simulink model "PneumaticsSystem"  (R2019b)
settings: configuration reference "ConfigSet_PneumaticsSystem_Reference" (kept outside this file)
PostLoadFcn:
  | set_up_test_model()
model workspace (MAT data in the model file):
  PAtm = 101300
  Prm_PneumaticsSystem : Simulink.Parameter (value not decoded)
  SampleTime = 0.01
symbols that are objects in the model workspace (value not decoded): Prm_PneumaticsSystem
undefined symbols (not defined in the file): AirSuspensionBogie1Deflated, AirSuspensionPressure, AirSuspensionPressureSwitch, AirSuspPressureDiff, AuxiliaryReservoirPressure, AuxiliaryReservoirPressureSwitch, BECU1BrakeNotApplied, BECU1BrakeNotReleased, BECU1CarLoadPressureLow, BECU1EmergencyBrakeFailure, BECU1LoadPressureLow, BECU1ServiceBrakeFailure, BECU2CarLoadPressureLow, BECU2EmergencyBrakeFailure, BECULowRPressure, Bogie, BrakeCylinderControlPressure, BrakeCylinderPressure, BrakeCylinderPressureGauge, BrakeCylinderPressureSwitch, BrakeReservoirPressure, BrakeReservoirPressureSwitch, HornHighPressureSwitch, HornLowPressureSwitch, MainReservoirPipePressure, MainReservoirPipePressureSwitch, MainReservoirPressure, MainReservoirPressureGauge, MainReservoirPressureSwitch, MaxAxles, MRPS_TractionCutout, ORDPressureSwitch, PantographCylinderPressure, ParkBrakePressure, ParkBrakePressureGauge, ParkBrakePressureSwitch, PS2, PS3, SandingSystemPressure, SandingSystemPressureSwitch, SRPressureGauge, VCBCylinderPressure, VCBPressureSwitch
libraries: PneumaticLib x56, simulink x50, LatchesLib x7, FiltersLib x4, TimersLib x3, MathOperationsLib x3, VectorOperationsLib x1, simulink_extras x1
(part 2 of 3)

== system PneumaticsSystem/PneumaticsPerVehicle/PneumaticsSystem/AuxiliarySystems/Horn ==
  ControlStates : Inport
  HornSupplyPressure : Inport  Port=2
  ElectricalSignals : Inport  Port=3
  Enable : EnablePort
  Bias : Bias  Bias=-PAtm
  Bus Creator : BusCreator  Inputs=2
  Bus Creator1 : BusCreator  Inputs=2
  Bus Selector : BusSelector  OutputSignals=HornLowIsolationCock,HornHighIsolationCock
  Bus Selector1 : BusSelector  OutputSignals=HornLowControl,HornHighControl,RemoteHornIsolate
  Data Type Conversion : DataTypeConversion
  Data Type Conversion1 : DataTypeConversion
  Enough Air : simulink/Logic and Bit Operations/Compare To Constant  relop=>  const=PressureSwitchON  OutDataTypeStr=boolean
  Enough Air1 : simulink/Logic and Bit Operations/Compare To Constant  relop=>  const=PressureSwitchON  OutDataTypeStr=boolean
  Gain : Gain
  Gain1 : Gain
  High Horn : simulink/Logic and Bit Operations/Compare To Constant  relop===  const=1  OutDataTypeStr=boolean
  Logical Operator : Logic  Inputs=3  AllPortsSameDT=off  OutDataTypeStr=boolean
  Logical Operator1 : Logic  Inputs=3  AllPortsSameDT=off  OutDataTypeStr=boolean
  Low Horn : simulink/Logic and Bit Operations/Compare To Constant  relop===  const=1  OutDataTypeStr=boolean
  NOT : Logic  Operator=NOT  AllPortsSameDT=off  OutDataTypeStr=boolean
  Product : Product
  Product1 : Product
  PressureSwitches : Outport
  AudioOut : Outport  Port=2
  wires:
  ControlStates/1 -> Bus Selector/1
  Bus Selector1/1 -> High Horn/1  "<HornLowControl>"
  Bias/1 -> Product1/2, Product/2
  Product/1 -> Enough Air/1
  High Horn/1 -> Logical Operator/1
  Low Horn/1 -> Logical Operator1/1
  Logical Operator/1 -> Data Type Conversion/1  "HornLowPressureSwitch"
  Logical Operator1/1 -> Data Type Conversion1/1  "HornHighPressureSwitch"
  Gain/1 -> Bus Creator/1  "HornLow"
  Gain1/1 -> Bus Creator/2  "HornHigh"
  Bus Creator/1 -> AudioOut/1
  Bus Creator1/1 -> PressureSwitches/1  "HornPressureSwitches"
  Data Type Conversion/1 -> Gain/1, Bus Creator1/1  "HornLowPressureSwitch"
  Data Type Conversion1/1 -> Gain1/1, Bus Creator1/2  "HornHighPressureSwitch"
  HornSupplyPressure/1 -> Bias/1
  ElectricalSignals/1 -> Bus Selector1/1
  Bus Selector/1 -> Product1/1  "<HornLowIsolationCock>"
  Bus Selector1/3 -> NOT/1  "<RemoteHornIsolate>"
  NOT/1 -> Logical Operator1/3, Logical Operator/3
  Bus Selector1/2 -> Low Horn/1  "<HornHighControl>"
  Product1/1 -> Enough Air1/1
  Enough Air1/1 -> Logical Operator/2
  Bus Selector/2 -> Product/1  "<HornHighIsolationCock>"
  Enough Air/1 -> Logical Operator1/2

== system PneumaticsSystem/PneumaticsPerVehicle/PneumaticsSystem/BogiePneumaticSystems/AirSuspensionSystem ==
  Faults : Inport
  ControlStates : Inport  Port=2
  PhysicalSignals : Inport  Port=3
  AirSuspensionSupplyPressure : Inport  Port=4
  Reset : Inport  Port=5
  Enable : EnablePort
  AirSuspensionPerBogie : Subsystem
  Bus Selector1 : BusSelector  OutputSignals=BogieSupportedMasses
  Bus Selector3 : BusSelector  OutputSignals=AirSuspensionSystemIsolationCockBogie1,AirSuspensionSystemIsolationCockBogie2,AirSuspensionSystemDrainCockBogie1,AirSuspensionSystemDrainCockBogie2
  Sum : Sum  Inputs=1
  Terminator : Terminator
  Vector Concatenate1 : Concatenate
  Vector Concatenate2 : Concatenate
  AirSuspensionPressure : Outport
  ASPressureSwitches : Outport  Port=2
  AirSuspPressure%Variation : Outport  Port=3
  ASRToAS : Outport  Port=4
  wires:
  ControlStates/1 -> Bus Selector3/1
  AirSuspensionPerBogie/1(AirSuspensionPressure) -> AirSuspensionPressure/1
  Bus Selector3/1 -> Vector Concatenate2/1  "<AirSuspensionSystemIsolationCockBogie1>"
  Reset/1 -> AirSuspensionPerBogie/5(Reset)
  Vector Concatenate1/1 -> AirSuspensionPerBogie/3(AirSuspensionDrainCock)
  PhysicalSignals/1 -> Bus Selector1/1
  Bus Selector3/2 -> Vector Concatenate2/2  "<AirSuspensionSystemIsolationCockBogie2>"
  Vector Concatenate2/1 -> AirSuspensionPerBogie/2(AirSuspensionIsolCock)
  AirSuspensionSupplyPressure/1 -> AirSuspensionPerBogie/1(AirSuspensionSupplyPressure)
  AirSuspensionPerBogie/3(AirSuspensionPressureSwitch) -> ASPressureSwitches/1
  Bus Selector1/1 -> AirSuspensionPerBogie/4(BogieSupportedMass)  "<BogieSupportedMasses>"
  Bus Selector3/3 -> Vector Concatenate1/1  "<AirSuspensionSystemDrainCockBogie1>"
  Bus Selector3/4 -> Vector Concatenate1/2  "<AirSuspensionSystemDrainCockBogie2>"
  AirSuspensionPerBogie/2(AirSuspensionValve) -> Terminator/1
  Faults/1 -> AirSuspensionPerBogie/6(Faults)
  AirSuspensionPerBogie/4(AirSuspPressure%Variation) -> AirSuspPressure%Variation/1
  AirSuspensionPerBogie/5(ASRToAS) -> Sum/1
  Sum/1 -> ASRToAS/1

== system PneumaticsSystem/PneumaticsPerVehicle/PneumaticsSystem/BogiePneumaticSystems/BogiePressureMapping ==
  BrakeControlPressures : Inport  Partition=on  PartitionDimension=1  PartitionWidth=1  PartitionOffset=0
  BrakeCylinderPressures : Inport  Port=2  Partition=on  PartitionDimension=1  PartitionWidth=2  PartitionOffset=0
  ParkBrakePressures : Inport  Port=3  Partition=on  PartitionDimension=1  PartitionWidth=1  PartitionOffset=0
  AirSuspensionPressures : Inport  Port=4  Partition=on  PartitionDimension=1  PartitionWidth=1  PartitionOffset=0
  SandingPressures : Inport  Port=5  Partition=on  PartitionDimension=1  PartitionWidth=1  PartitionOffset=0
  AirSuspPressure%Variation : Inport  Port=6  Partition=on  PartitionDimension=1  PartitionWidth=1  PartitionOffset=0
  Bus Assignment : BusAssignment  AssignedSignals=BrakeCylinderControlPressure,BrakeCylinderPressure,ParkBrakePressure,SandingSystemPressure,AirSuspensionPressure,AirSuspPressureDiff
  Constant : Constant  Value=0  OutDataTypeStr=Bus: BD_PneumaticsSystem_Out_Vehicle_Debug_Bogie
  For Each : ForEach  DisableCoverage=on
  BogiePressures : Outport  ConcatenationDimension=1
  wires:
  BrakeCylinderPressures/1 -> Bus Assignment/3
  Constant/1 -> Bus Assignment/1
  Bus Assignment/1 -> BogiePressures/1  "Debug"
  ParkBrakePressures/1 -> Bus Assignment/4
  AirSuspensionPressures/1 -> Bus Assignment/6
  SandingPressures/1 -> Bus Assignment/5
  BrakeControlPressures/1 -> Bus Assignment/2
  AirSuspPressure%Variation/1 -> Bus Assignment/7

== system PneumaticsSystem/PneumaticsPerVehicle/PneumaticsSystem/BogiePneumaticSystems/BogiePressureSwitchesMapping ==
  BrakeCylinderPressureSwitches : Inport  Partition=on  PartitionDimension=1  PartitionWidth=1  PartitionOffset=0
  ParkBrakePressureSwitches : Inport  Port=2  Partition=on  PartitionDimension=1  PartitionWidth=1  PartitionOffset=0
  AirSuspensionPressureSwitches : Inport  Port=3  Partition=on  PartitionDimension=1  PartitionWidth=1  PartitionOffset=0
  SandingPressureSwitches : Inport  Port=4  Partition=on  PartitionDimension=1  PartitionWidth=1  PartitionOffset=0
  Bus Assignment : BusAssignment  AssignedSignals=BrakeCylinderPressureSwitch,ParkBrakePressureSwitch,AirSuspensionPressureSwitch,SandingSystemPressureSwitch
  Constant : Constant  Value=0  OutDataTypeStr=Bus: BD_PneumaticsSystem_Out_Vehicle_Switches_Bogie
  For Each : ForEach  DisableCoverage=on
  BogiePressureSwitches : Outport  ConcatenationDimension=1
  wires:
  SandingPressureSwitches/1 -> Bus Assignment/5
  AirSuspensionPressureSwitches/1 -> Bus Assignment/4
  Bus Assignment/1 -> BogiePressureSwitches/1
  Constant/1 -> Bus Assignment/1
  ParkBrakePressureSwitches/1 -> Bus Assignment/3
  BrakeCylinderPressureSwitches/1 -> Bus Assignment/2

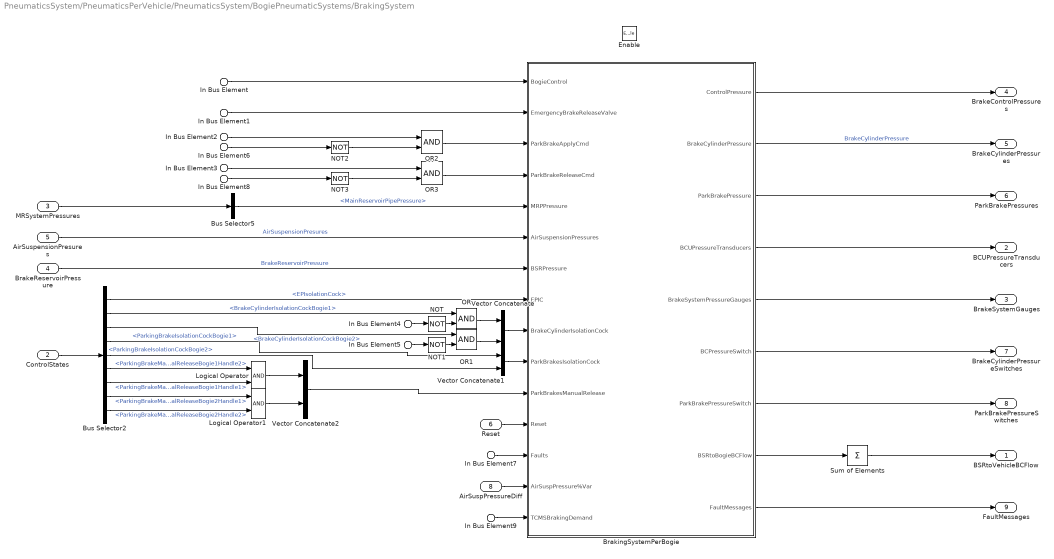
== system PneumaticsSystem/PneumaticsPerVehicle/PneumaticsSystem/BogiePneumaticSystems/BrakingSystem ==
  In Bus Element : Inport  PortName=ElectricalSignals  Element=BogieControl
  In Bus Element1 : Inport  PortName=ElectricalSignals  Element=NoEmergencyBrakeValve
  In Bus Element2 : Inport  PortName=ElectricalSignals  Element=ParkingBrakeApplyCmd
  In Bus Element3 : Inport  PortName=ElectricalSignals  Element=ParkingBrakeReleaseCmd
  In Bus Element9 : Inport  PortName=ElectricalSignals  Element=TCMSBrakingDemand
  In Bus Element4 : Inport  PortName=ElectricalSignals  Element=RemoteMagnetValve1
  In Bus Element5 : Inport  PortName=ElectricalSignals  Element=RemoteMagnetValve2
  ControlStates : Inport  Port=2
  MRSystemPressures : Inport  Port=3
  BrakeReservoirPressure : Inport  Port=4
  AirSuspensionPresures : Inport  Port=5
  Reset : Inport  Port=6
  In Bus Element7 : Inport  Port=7  PortName=PneumaticsFaults
  In Bus Element6 : Inport  Port=7  PortName=PneumaticsFaults  Element=ParkingBrakeApplicationFailure
  In Bus Element8 : Inport  Port=7  PortName=PneumaticsFaults  Element=ParkingBrakeReleaseFailure
  AirSuspPressureDiff : Inport  Port=8
  Enable : EnablePort
  BrakingSystemPerBogie : Subsystem
  Bus Selector2 : BusSelector  OutputSignals=EPIsolationCock,BrakeCylinderIsolationCockBogie1,BrakeCylinderIsolationCockBogie2,ParkingBrakeIsolationCockBogie1,ParkingBrakeIsolationCockBogie2,ParkingBrakeManualReleaseBogie1Handle2,ParkingBrakeManualReleaseBogie1Handle1,ParkingBrakeManualReleaseBogie2Handle1,ParkingBrakeManualReleaseBogie2Handle2
  Bus Selector5 : BusSelector  OutputSignals=MainReservoirPipePressure
  Logical Operator : Logic  AllPortsSameDT=off  OutDataTypeStr=boolean
  Logical Operator1 : Logic  AllPortsSameDT=off  OutDataTypeStr=boolean
  NOT{,1..3} (4 alike) : Logic  Operator=NOT  AllPortsSameDT=off  OutDataTypeStr=boolean
  OR{,1..3} (4 alike) : Logic  AllPortsSameDT=off  OutDataTypeStr=boolean
  Sum of Elements : Sum  Inputs=+
  Vector Concatenate : Concatenate
  Vector Concatenate1 : Concatenate
  Vector Concatenate2 : Concatenate
  BSRtoVehicleBCFlow : Outport
  BCUPressureTransducers : Outport  Port=2
  BrakeSystemGauges : Outport  Port=3
  BrakeControlPressures : Outport  Port=4
  BrakeCylinderPressures : Outport  Port=5
  ParkBrakePressures : Outport  Port=6
  BrakeCylinderPressureSwitches : Outport  Port=7
  ParkBrakePressureSwitches : Outport  Port=8
  FaultMessages : Outport  Port=9
  wires:
  BrakingSystemPerBogie/1(ControlPressure) -> BrakeControlPressures/1
  In Bus Element/1 -> BrakingSystemPerBogie/1(BogieControl)
  In Bus Element1/1 -> BrakingSystemPerBogie/2(EmergencyBrakeReleaseValve)
  BrakeReservoirPressure/1 -> BrakingSystemPerBogie/7(BSRPressure)  "BrakeReservoirPressure"
  ControlStates/1 -> Bus Selector2/1
  AirSuspensionPresures/1 -> BrakingSystemPerBogie/6("AirSuspensionPressures ")  "AirSuspensionPresures"
  BrakingSystemPerBogie/2(BrakeCylinderPressure) -> BrakeCylinderPressures/1  "BrakeCylinderPressure"
  BrakingSystemPerBogie/8(BSRtoBogieBCFlow) -> Sum of Elements/1
  Bus Selector5/1 -> BrakingSystemPerBogie/5(MRPPressure)  "<MainReservoirPipePressure>"
  BrakingSystemPerBogie/5(BrakeSystemPressureGauges) -> BrakeSystemGauges/1
  BrakingSystemPerBogie/7(ParkBrakePressureSwitch) -> ParkBrakePressureSwitches/1
  BrakingSystemPerBogie/3(ParkBrakePressure) -> ParkBrakePressures/1
  BrakingSystemPerBogie/4(BCUPressureTransducers) -> BCUPressureTransducers/1
  MRSystemPressures/1 -> Bus Selector5/1
  BrakingSystemPerBogie/6(BCPressureSwitch) -> BrakeCylinderPressureSwitches/1
  Reset/1 -> BrakingSystemPerBogie/12(Reset)
  Sum of Elements/1 -> BSRtoVehicleBCFlow/1
  Bus Selector2/6 -> Logical Operator/1  "<ParkingBrakeManualReleaseBogie1Handle2>"
  Bus Selector2/7 -> Logical Operator/2  "<ParkingBrakeManualReleaseBogie1Handle1>"
  Vector Concatenate2/1 -> BrakingSystemPerBogie/11(ParkBrakesManualRelease)
  In Bus Element2/1 -> OR2/1
  In Bus Element3/1 -> OR3/1
  Bus Selector2/8 -> Logical Operator1/1  "<ParkingBrakeManualReleaseBogie2Handle1>"
  Bus Selector2/9 -> Logical Operator1/2  "<ParkingBrakeManualReleaseBogie2Handle2>"
  Logical Operator/1 -> Vector Concatenate2/1
  Logical Operator1/1 -> Vector Concatenate2/2
  In Bus Element7/1 -> BrakingSystemPerBogie/13(Faults)
  OR2/1 -> BrakingSystemPerBogie/3(ParkBrakeApplyCmd)
  OR3/1 -> BrakingSystemPerBogie/4(ParkBrakeReleaseCmd)
  NOT2/1 -> OR2/2
  In Bus Element6/1 -> NOT2/1
  NOT3/1 -> OR3/2
  In Bus Element8/1 -> NOT3/1
  BrakingSystemPerBogie/9(FaultMessages) -> FaultMessages/1
  AirSuspPressureDiff/1 -> BrakingSystemPerBogie/14(AirSuspPressure%Var)
  Bus Selector2/1 -> BrakingSystemPerBogie/8(EPIC)  "<EPIsolationCock>"
  In Bus Element9/1 -> BrakingSystemPerBogie/15(TCMSBrakingDemand)
  Vector Concatenate/1 -> BrakingSystemPerBogie/9(BrakeCylinderIsolationCock)
  Bus Selector2/4 -> Vector Concatenate1/1  "<ParkingBrakeIsolationCockBogie1>"
  OR/1 -> Vector Concatenate/1
  NOT1/1 -> OR1/2
  In Bus Element5/1 -> NOT1/1
  Bus Selector2/3 -> OR1/1  "<BrakeCylinderIsolationCockBogie2>"
  Bus Selector2/5 -> Vector Concatenate1/2  "<ParkingBrakeIsolationCockBogie2>"
  In Bus Element4/1 -> NOT/1
  NOT/1 -> OR/2
  OR1/1 -> Vector Concatenate/2
  Bus Selector2/2 -> OR/1  "<BrakeCylinderIsolationCockBogie1>"
  Vector Concatenate1/1 -> BrakingSystemPerBogie/10(ParkBrakesIsolationCock)

== system PneumaticsSystem/PneumaticsPerVehicle/PneumaticsSystem/BogiePneumaticSystems/SandingSystem ==
  ElectricalSignals : Inport
  ControlStates : Inport  Port=2
  SandingSystemSupplyPressure : Inport  Port=3
  Enable : EnablePort
  Bus Selector1 : BusSelector  OutputSignals=SandingSystemIsolationCockBogie1,SandingSystemIsolationCockBogie2
  Bus Selector2 : BusSelector  OutputSignals=SandingValve
  SandingSystemPerBogie : Subsystem
  Vector Concatenate : Concatenate
  SandingPressures : Outport
  SandingPressureSwitches : Outport  Port=2
  wires:
  ElectricalSignals/1 -> Bus Selector2/1
  ControlStates/1 -> Bus Selector1/1
  Bus Selector1/1 -> Vector Concatenate/1  "<SandingSystemIsolationCockBogie1>"
  Bus Selector1/2 -> Vector Concatenate/2  "<SandingSystemIsolationCockBogie2>"
  Vector Concatenate/1 -> SandingSystemPerBogie/1(SandingSystemIsolationCock)  "SandingSystemIsolationCock"
  SandingSystemSupplyPressure/1 -> SandingSystemPerBogie/2(SandingSystemSupplyPressure)
  Bus Selector2/1 -> SandingSystemPerBogie/3(SandingValve)  "<SandingValve>"
  SandingSystemPerBogie/1(SandingPressure) -> SandingPressures/1
  SandingSystemPerBogie/2(SandingPressureSwitch) -> SandingPressureSwitches/1

== system PneumaticsSystem/PneumaticsPerVehicle/PneumaticsSystem/BrakeReservoirSystem/BrakeSupplyReservoir ==
  MRPPressure : Inport
  BSRIsolCock : Inport  Port=2
  BSRDrainCock : Inport  Port=3
  BSRtoBCFlow : Inport  Port=4
  LowRPress : Inport  Port=5
  Reset : Inport  Port=6
  Preset : Inport  Port=7
  PresetVal : Inport  Port=8
  Enable : EnablePort
  BSRPressureSwitch.05 : PneumaticLib/Pressure Switch  OnSwitchValue=PressureSwitchON  OffSwitchValue=PressureSwitchOFF  OnOutputValue=1  OffOutputValue=0  InitOn=on
      settings: SourceProductName=Train Library
  Bias : Bias  Bias=-PAtm
  BrakeSupplyReservoir : PneumaticLib/Limited Air Pressure Vessel  resetPrs=ResetPressure + PAtm
      settings: SourceProductName=Pneumatic
  Constant : Constant  Value=PAtm + MaxPressure
  Display : Display
  FlowCalc : Subsystem
  Terminator : Terminator
  Unit Delay : UnitDelay  SampleTime=-1  HasFrameUpgradeWarning=on
  pAtm : Constant  Value=PAtm
  pAtm2 : Constant  Value=Volume
  BSRPressure : Outport
  BSRPressureSwitch : Outport  Port=2
  MRPToBSR : Outport  Port=3
  BSRPressureGauge : Outport  Port=4
  wires:
  pAtm2/1 -> BrakeSupplyReservoir/2
  pAtm/1 -> BrakeSupplyReservoir/4
  Reset/1 -> BrakeSupplyReservoir/5
  Unit Delay/1 -> FlowCalc/2(BSRPressure)
  MRPPressure/1 -> FlowCalc/1(MRPressure)
  Constant/1 -> BrakeSupplyReservoir/3
  FlowCalc/2(Flow) -> BrakeSupplyReservoir/1
  BrakeSupplyReservoir/1 -> BSRPressure/1, Bias/1, Unit Delay/1
  BrakeSupplyReservoir/2 -> Terminator/1
  BSRIsolCock/1 -> FlowCalc/3(BSRIsolCock)
  BSRtoBCFlow/1 -> FlowCalc/5(BSRtoBCFlow)
  BSRDrainCock/1 -> FlowCalc/4(BSRDrainCock)
  BSRPressureSwitch.05/1 -> BSRPressureSwitch/1  "BrakeReservoirPressureSwitch"
  Bias/1 -> BSRPressureGauge/1, Display/1, BSRPressureSwitch.05/1
  PresetVal/1 -> BrakeSupplyReservoir/7
  Preset/1 -> BrakeSupplyReservoir/6
  LowRPress/1 -> FlowCalc/6(Fault)
  FlowCalc/1(MRPToBSR) -> MRPToBSR/1

== system PneumaticsSystem/PneumaticsPerVehicle/PneumaticsSystem/GaugesMapping/Subsystem ==
  BCPressure : Inport  Partition=on  PartitionDimension=1  PartitionWidth=1  PartitionOffset=0
  Bus Assignment1 : BusAssignment  AssignedSignals=BrakeCylinderPressureGauge,ParkBrakePressureGauge
  Bus Selector : BusSelector  OutputSignals=BrakeCylinderPressureGauge,ParkBrakePressureGauge
  Constant1 : Constant  Value=0  OutDataTypeStr=Bus: BD_PneumaticsSystem_Out_Vehicle_Gauges_Bogie
  For Each : ForEach  DisableCoverage=on
  Bogie : Outport  ConcatenationDimension=1
  wires:
  Constant1/1 -> Bus Assignment1/1
  Bus Assignment1/1 -> Bogie/1  "Bogie"
  Bus Selector/1 -> Bus Assignment1/2  "<BrakeCylinderPressureGauge>"
  BCPressure/1 -> Bus Selector/1
  Bus Selector/2 -> Bus Assignment1/3  "<ParkBrakePressureGauge>"

== system PneumaticsSystem/PneumaticsPerVehicle/PneumaticsSystem/MainReservoirSystem/MainReservoir ==
  note: This pressure switch is not a part of
      | schematics and not used anywhere.
  CompressorRunning : Inport
  AirSupplyIsolationCock : Inport  Port=2
  MainReservoirIsolationCock : Inport  Port=3
  MainReservoirDrainCock : Inport  Port=4
  MRPPressure : Inport  Port=5
  Coupled : Inport  Port=6
  Reset : Inport  Port=7
  Enable : EnablePort
  Bias : Bias  Bias=-PAtm
  Constant : Constant  Value=PAtm + MaxPressure
  Display : Display
  FlowCalc : Subsystem
  Ground2 : Ground
  MRPressureSwitch.06 : PneumaticLib/Pressure Switch  OnSwitchValue=PressureSwitchON  OffSwitchValue=PressureSwitchOFF  OnOutputValue=1  OffOutputValue=0  InitOn=on
      settings: SourceProductName=Train Library
  MainReservoir : PneumaticLib/Limited Air Pressure Vessel  resetPrs=ResetPressure + PAtm
      settings: SourceProductName=Pneumatic
  Terminator : Terminator
  Unit Delay : UnitDelay  SampleTime=-1  HasFrameUpgradeWarning=on
  Vol : Constant  Value=Volume
  pAtm : Constant  Value=PAtm
  MRPressure : Outport
  MRPressureSwitch : Outport  Port=2
  MRPToMRFlow : Outport  Port=3
  wires:
  MainReservoir/2 -> Terminator/1
  FlowCalc/2(Flow) -> MainReservoir/1
  MainReservoir/1 -> MRPressure/1, Bias/1, Unit Delay/1  "MainReservoirPressure"
  Constant/1 -> MainReservoir/3
  MRPPressure/1 -> FlowCalc/6(MRPPressure)
  Unit Delay/1 -> FlowCalc/7(MRPressure)
  Reset/1 -> MainReservoir/5
  pAtm/1 -> MainReservoir/4
  Ground2/1 -> MainReservoir/6, MainReservoir/7
  Vol/1 -> MainReservoir/2
  CompressorRunning/1 -> FlowCalc/1(CompressorRunning)
  AirSupplyIsolationCock/1 -> FlowCalc/2(AirSupplyIsolCock)
  MainReservoirIsolationCock/1 -> FlowCalc/3(MRIsolCock)
  MainReservoirDrainCock/1 -> FlowCalc/4(MRDrainCock)
  MRPressureSwitch.06/1 -> MRPressureSwitch/1  "MainReservoirPressureSwitch"
  Bias/1 -> MRPressureSwitch.06/1, Display/1
  FlowCalc/1(MRPToMRFlow) -> MRPToMRFlow/1
  Coupled/1 -> FlowCalc/5(Coupled)

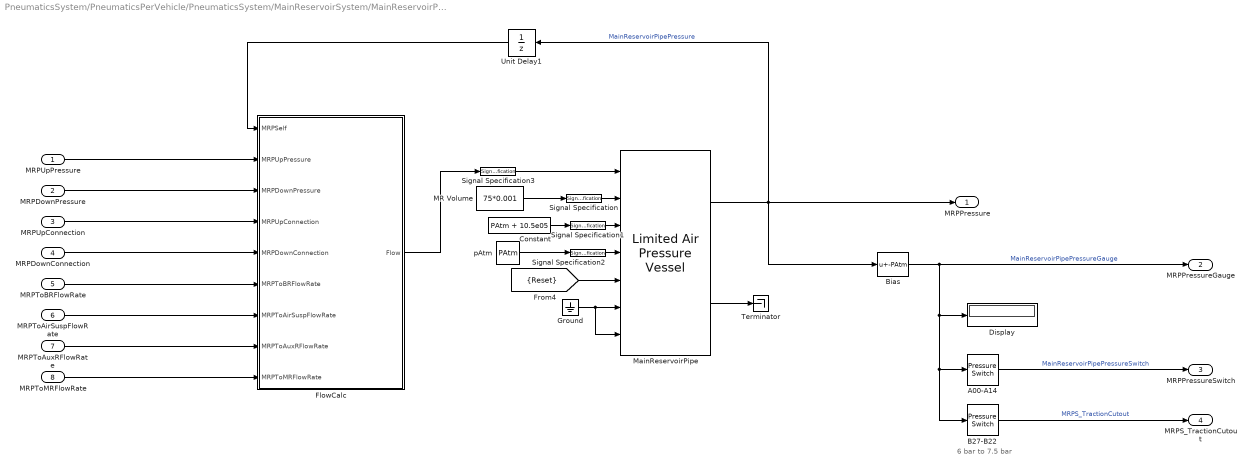
== system PneumaticsSystem/PneumaticsPerVehicle/PneumaticsSystem/MainReservoirSystem/MainReservoirPipe ==
  note: 6 bar to 7.5 bar
  MRPUpPressure : Inport
  MRPDownPressure : Inport  Port=2
  MRPUpConnection : Inport  Port=3
  MRPDownConnection : Inport  Port=4
  MRPToBRFlowRate : Inport  Port=5
  MRPToAirSuspFlowRate : Inport  Port=6
  MRPToAuxRFlowRate : Inport  Port=7
  MRPToMRFlowRate : Inport  Port=8
  A00-A14 : PneumaticLib/Pressure Switch  OnSwitchValue=PressureSwitchON  OffSwitchValue=PressureSwitchOFF  OnOutputValue=1  OffOutputValue=0  InitOn=on
      settings: SourceProductName=Train Library
  B27-B22 : PneumaticLib/Pressure Switch  OnSwitchValue=7e5  OffSwitchValue=6e5  OnOutputValue=1  OffOutputValue=0  InitOn=on
      settings: SourceProductName=Train Library
  Bias : Bias  Bias=-PAtm
  Constant : Constant  Value=PAtm + 10.5e05
  Display : Display
  FlowCalc : Subsystem
  Ground : Ground
  MR Volume : Constant  Value=75*0.001
  MainReservoirPipe : PneumaticLib/Limited Air Pressure Vessel  resetPrs=ResetPressure + PAtm
      settings: SourceProductName=Pneumatic
  Signal Specification : SignalSpecification  Unit=m^3
  Signal Specification1 : SignalSpecification  Unit=Pa
  Signal Specification2 : SignalSpecification  Unit=Pa
  Signal Specification3 : SignalSpecification  Unit=kg/s
  Terminator : Terminator
  Unit Delay1 : UnitDelay  SampleTime=-1  HasFrameUpgradeWarning=on
  pAtm : Constant  Value=PAtm
  MRPPressure : Outport  VectorParamsAs1DForOutWhenUnconnected=off
  MRPPressureGauge : Outport  Port=2
  MRPPressureSwitch : Outport  Port=3
  MRPS_TractionCutout : Outport  Port=4
  wires:
  MRPToBRFlowRate/1 -> FlowCalc/6(MRPToBRFlowRate)
  [Reset] -> MainReservoirPipe/5
  MRPToAirSuspFlowRate/1 -> FlowCalc/7(MRPToAirSuspFlowRate)
  Unit Delay1/1 -> FlowCalc/1(MRPSelf)
  Signal Specification2/1 -> MainReservoirPipe/4
  MRPToMRFlowRate/1 -> FlowCalc/9(MRPToMRFlowRate)
  Signal Specification/1 -> MainReservoirPipe/2
  MainReservoirPipe/2 -> Terminator/1
  Signal Specification3/1 -> MainReservoirPipe/1
  pAtm/1 -> Signal Specification2/1
  MR Volume/1 -> Signal Specification/1
  Constant/1 -> Signal Specification1/1
  FlowCalc/1(Flow) -> Signal Specification3/1
  MRPDownPressure/1 -> FlowCalc/3(MRPDownPressure)
  MRPUpPressure/1 -> FlowCalc/2(MRPUpPressure)
  MRPDownConnection/1 -> FlowCalc/5(MRPDownConnection)
  Signal Specification1/1 -> MainReservoirPipe/3
  MRPUpConnection/1 -> FlowCalc/4(MRPUpConnection)
  MainReservoirPipe/1 -> Bias/1, Unit Delay1/1, MRPPressure/1  "MainReservoirPipePressure"
  A00-A14/1 -> MRPPressureSwitch/1  "MainReservoirPipePressureSwitch"
  Bias/1 -> A00-A14/1, B27-B22/1, Display/1, MRPPressureGauge/1  "MainReservoirPipePressureGauge"
  B27-B22/1 -> MRPS_TractionCutout/1  "MRPS_TractionCutout"
  MRPToAuxRFlowRate/1 -> FlowCalc/8(MRPToAuxRFlowRate)
  Ground/1 -> MainReservoirPipe/7, MainReservoirPipe/6

== system PneumaticsSystem/PneumaticsPerVehicle/PneumaticsSystem/ASReservoir/Air SuspensionReservoir/FlowCalc ==
  MRPressure : Inport
  ASRPressure : Inport  Port=2
  ASRIsolCock : Inport  Port=3
  ASRDrainCock : Inport  Port=4
  ASFlow : Inport  Port=5
  Add : Sum  Inputs=+---
  BSR Charge : PneumaticLib/SS One Way Valve  d=0.015  p_deadband=1000
      settings: SourceProductName=Train Library
  BSR Vent Drain : PneumaticLib/SS One Way Valve  d=0.015  p_deadband=1000
      settings: SourceProductName=Train Library
  BSR Vent IC : PneumaticLib/SS One Way Valve  d=0.015  p_deadband=1000
      settings: SourceProductName=Train Library
  Compare To Constant : simulink/Logic and Bit Operations/Compare To Constant  relop=>=  const=780000  OutDataTypeStr=boolean
  Constant : Constant  Value=PAtm
  Logical Operator1 : Logic  Operator=NOT  AllPortsSameDT=off  OutDataTypeStr=boolean
  Logical Operator2 : Logic  Operator=NOT  AllPortsSameDT=off  OutDataTypeStr=boolean
  Logical Operator3 : Logic  Operator=OR  AllPortsSameDT=off  OutDataTypeStr=boolean
  Terminator : Terminator
  Terminator1 : Terminator
  Terminator4 : Terminator
  MRPToASR : Outport
  Flow : Outport  Port=2
  wires:
  Logical Operator2/1 -> BSR Vent Drain/3
  ASFlow/1 -> Add/4
  ASRDrainCock/1 -> Logical Operator2/1
  BSR Vent Drain/1 -> Add/3
  BSR Vent Drain/2 -> Terminator4/1
  ASRPressure/1 -> Compare To Constant/1, BSR Charge/2, BSR Vent IC/1, BSR Vent Drain/1
  Logical Operator1/1 -> Logical Operator3/1
  ASRIsolCock/1 -> Logical Operator1/1, BSR Vent IC/3
  Constant/1 -> BSR Vent Drain/2, BSR Vent IC/2
  MRPressure/1 -> BSR Charge/1
  BSR Vent IC/1 -> Add/2
  BSR Vent IC/2 -> Terminator1/1
  BSR Charge/2 -> Terminator/1
  Add/1 -> Flow/1
  BSR Charge/1 -> MRPToASR/1, Add/1
  Logical Operator3/1 -> BSR Charge/3
  Compare To Constant/1 -> Logical Operator3/2

== system PneumaticsSystem/PneumaticsPerVehicle/PneumaticsSystem/AuxiliarySystems/AuxSystem/AuxReservoir ==
  CompressorRunning : Inport
  MRPPressure : Inport  Port=2
  AuxCompIsolCock : Inport  Port=3
  ARIsolCock : Inport  Port=4
  ARDrainCock : Inport  Port=5
  ARtoPCandVCBFlow : Inport  Port=6
  Reset : Inport  Port=7
  ARPressureSwitch.12 : PneumaticLib/Pressure Switch  OnSwitchValue=PressureSwitchON  OffSwitchValue=PressureSwitchOFF  OnOutputValue=1  OffOutputValue=0  InitOn=on
      settings: SourceProductName=Train Library
  AuxReservoir : PneumaticLib/Limited Air Pressure Vessel  resetPrs=ResetPressure + PAtm
      settings: SourceProductName=Pneumatic
  Bias : Bias  Bias=-PAtm
  Constant : Constant  Value=PAtm + MaxPressure
  Display : Display
  FlowCalc : Subsystem
  Ground2 : Ground
  Terminator : Terminator
  Unit Delay : UnitDelay  SampleTime=-1  HasFrameUpgradeWarning=on
  pAtm : Constant  Value=PAtm
  pAtm2 : Constant  Value=Volume
  ARPressure : Outport
  ARPressureSwitch : Outport  Port=2
  MRPToAuxR : Outport  Port=3
  wires:
  ARtoPCandVCBFlow/1 -> FlowCalc/7(ARtoPCFlow)  "ARtoPCFlow"
  ARDrainCock/1 -> FlowCalc/6(ARDrainCock)  "ARDrainCock"
  AuxCompIsolCock/1 -> FlowCalc/4(AuxCompIsolCock)
  AuxReservoir/2 -> Terminator/1
  FlowCalc/2(Flow) -> AuxReservoir/1  "ARFlow"
  AuxReservoir/1 -> Bias/1, ARPressure/1, Unit Delay/1  "AuxiliaryReservoirPressure"
  Constant/1 -> AuxReservoir/3
  pAtm/1 -> AuxReservoir/4
  Ground2/1 -> AuxReservoir/7, AuxReservoir/6
  pAtm2/1 -> AuxReservoir/2
  CompressorRunning/1 -> FlowCalc/1(CompressorRunning)
  ARPressureSwitch.12/1 -> ARPressureSwitch/1  "AuxiliaryReservoirPressureSwitch"
  Bias/1 -> ARPressureSwitch.12/1, Display/1
  Reset/1 -> AuxReservoir/5
  ARIsolCock/1 -> FlowCalc/5(ARIsolCock)
  Unit Delay/1 -> FlowCalc/3(ARPressure)
  MRPPressure/1 -> FlowCalc/2(MRPPressure)
  FlowCalc/1(MRPToAuxR) -> MRPToAuxR/1

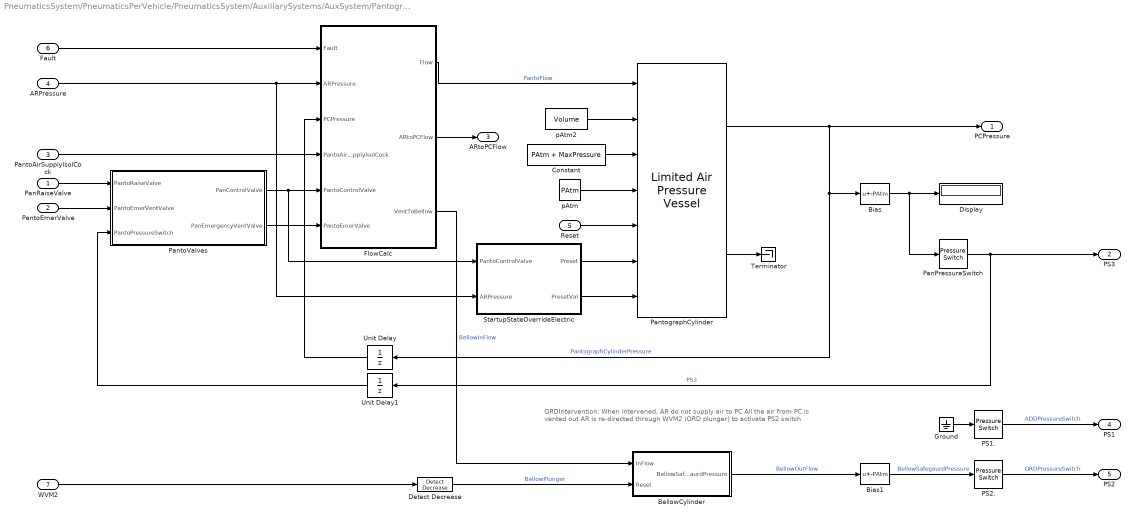
== system PneumaticsSystem/PneumaticsPerVehicle/PneumaticsSystem/AuxiliarySystems/AuxSystem/Pantograph ==
  note: ORDIntervention:
      | When intervened, AR do not supply air to PC
      | All the air from PC is vented out
      | AR is re-directed through WVM2 (ORD plunger) to activate PS2 switch
  PanRaiseValve : Inport
  PantoEmerValve : Inport  Port=2
  PantoAirSupplyIsolCock : Inport  Port=3
  ARPressure : Inport  Port=4
  Reset : Inport  Port=5
  Fault : Inport  Port=6
  WVM2 : Inport  Port=7
  BellowCylinder : Subsystem
  Bias : Bias  Bias=-PAtm
  Bias1 : Bias  Bias=-PAtm
  Constant : Constant  Value=PAtm + MaxPressure
  Detect Decrease : simulink/Logic and Bit Operations/Detect Decrease  vinit=0.0  OutDataTypeStr=boolean
  Display : Display
  FlowCalc : Subsystem
  Ground : Ground
  PS1. : PneumaticLib/Pressure Switch  OnSwitchValue=PressureSwitchON  OffSwitchValue=PressureSwitchOFF  OnOutputValue=1  OffOutputValue=0  InitOn=on
      settings: SourceProductName=Train Library
  PS2. : PneumaticLib/Pressure Switch  OnSwitchValue=ORDPressureSwitchON  OffSwitchValue=ORDPressureSwitchOFF  OnOutputValue=1  OffOutputValue=0  InitOn=on
      settings: SourceProductName=Train Library
  PanPressureSwitch : PneumaticLib/Pressure Switch  OnSwitchValue=PressureSwitchON  OffSwitchValue=PressureSwitchOFF  OnOutputValue=1  OffOutputValue=0  InitOn=on
      settings: SourceProductName=Train Library
  PantoValves : Subsystem
  PantographCylinder : PneumaticLib/Limited Air Pressure Vessel  resetPrs=PAtm + ResetPressure
      settings: SourceProductName=Pneumatic
  StartupStateOverrideElectric : Subsystem
  Terminator : Terminator
  Unit Delay : UnitDelay  SampleTime=-1  HasFrameUpgradeWarning=on
  Unit Delay1 : UnitDelay  SampleTime=-1  HasFrameUpgradeWarning=on
  pAtm : Constant  Value=PAtm
  pAtm2 : Constant  Value=Volume
  PCPressure : Outport
  PS3 : Outport  Port=2
  ARtoPCFlow : Outport  Port=3
  PS1 : Outport  Port=4
  PS2 : Outport  Port=5
  wires:
  PanPressureSwitch/1 -> Unit Delay1/1, PS3/1  "PS3"
  pAtm2/1 -> PantographCylinder/2
  pAtm/1 -> PantographCylinder/4
  Unit Delay/1 -> FlowCalc/3(PCPressure)
  ARPressure/1 -> FlowCalc/2(ARPressure), StartupStateOverrideElectric/2(ARPressure)
  Constant/1 -> PantographCylinder/3
  FlowCalc/1(Flow) -> PantographCylinder/1  "PantoFlow"
  PantographCylinder/2 -> Terminator/1
  PantoAirSupplyIsolCock/1 -> FlowCalc/4(PantoAirSupplyIsolCock)
  FlowCalc/2(ARtoPCFlow) -> ARtoPCFlow/1
  PanRaiseValve/1 -> PantoValves/1(PantoRaiseValve)
  PantoValves/1(PanControlValve) -> FlowCalc/5(PantoControlValve), StartupStateOverrideElectric/1(PantoControlValve)
  PantoValves/2(PanEmergencyVentValve) -> FlowCalc/6(PantoEmerValve)
  PantoEmerValve/1 -> PantoValves/2(PantoEmerVentValve)
  Reset/1 -> PantographCylinder/5
  StartupStateOverrideElectric/1(Preset) -> PantographCylinder/6
  StartupStateOverrideElectric/2(PresetVal) -> PantographCylinder/7
  Unit Delay1/1 -> PantoValves/3(PantoPressureSwitch)
  PantographCylinder/1 -> PCPressure/1, Unit Delay/1, Bias/1  "PantographCylinderPressure"
  Fault/1 -> FlowCalc/1(Fault)
  PS2./1 -> PS2/1  "ORDPressureSwitch"
  PS1./1 -> PS1/1  "ADDPressureSwitch"
  Ground/1 -> PS1./1
  Bias/1 -> Display/1, PanPressureSwitch/1
  Bias1/1 -> PS2./1  "BellowSafegaurdPressure"
  WVM2/1 -> Detect Decrease/1
  BellowCylinder/1(BellowSafegaurdPressure) -> Bias1/1  "BellowOutFlow"
  FlowCalc/3(VentToBellow) -> BellowCylinder/1(InFlow)  "BellowInFlow"
  Detect Decrease/1 -> BellowCylinder/2(Reset)  "BellowPlunger"

== system PneumaticsSystem/PneumaticsPerVehicle/PneumaticsSystem/AuxiliarySystems/AuxSystem/VCB ==
  ARPressure : Inport
  Reset1 : Inport  Port=2
  VCBC : Inport  Port=3
  VCBIsolationCock : Inport  Port=4
  Bias : Bias  Bias=-PAtm
  Constant : Constant  Value=PAtm + MaxPressure
  Ground : Ground
  Subsystem : Subsystem
  Terminator1 : Terminator
  Unit Delay1 : UnitDelay  SampleTime=-1  HasFrameUpgradeWarning=on
  VCBCylinder : PneumaticLib/Limited Air Pressure Vessel  resetPrs=PAtm + ResetPressure
      settings: SourceProductName=Pneumatic
  VCBPressureSwitch1 : PneumaticLib/Pressure Switch  OnSwitchValue=PressureSwitchON  OffSwitchValue=PressureSwitchOFF  OnOutputValue=1  OffOutputValue=0  InitOn=on
      settings: SourceProductName=Train Library
  pAtm : Constant  Value=PAtm
  pAtm2 : Constant  Value=Volume
  VCBCylinderPressure : Outport
  VCBPressureSwitch : Outport  Port=2
  ARtoVCB : Outport  Port=3
  wires:
  Ground/1 -> VCBCylinder/6, VCBCylinder/7
  Reset1/1 -> VCBCylinder/5
  pAtm/1 -> VCBCylinder/4
  VCBCylinder/2 -> Terminator1/1
  pAtm2/1 -> VCBCylinder/2
  Constant/1 -> VCBCylinder/3
  VCBPressureSwitch1/1 -> VCBPressureSwitch/1  "VCBPressureSwitch"
  VCBCylinder/1 -> VCBCylinderPressure/1, Unit Delay1/1, Bias/1  "VCBCylinderPressure"
  Subsystem/2(Flow) -> VCBCylinder/1
  ARPressure/1 -> Subsystem/1(ARP)
  Unit Delay1/1 -> Subsystem/2(VCBP)
  Subsystem/1(ARToVCB) -> ARtoVCB/1
  Bias/1 -> VCBPressureSwitch1/1
  VCBC/1 -> Subsystem/3(VCBCloseCmd)
  VCBIsolationCock/1 -> Subsystem/4(VCBIsolationCock)

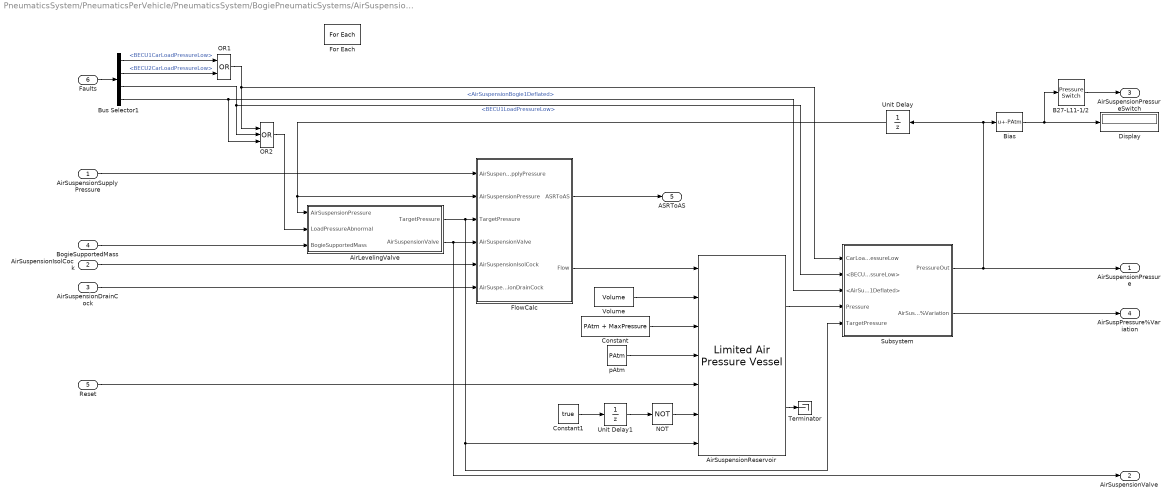
== system PneumaticsSystem/PneumaticsPerVehicle/PneumaticsSystem/BogiePneumaticSystems/AirSuspensionSystem/AirSuspensionPerBogie ==
  AirSuspensionSupplyPressure : Inport
  AirSuspensionIsolCock : Inport  Port=2  Partition=on  PartitionDimension=1  PartitionWidth=1  PartitionOffset=0
  AirSuspensionDrainCock : Inport  Port=3  Partition=on  PartitionDimension=1  PartitionWidth=1  PartitionOffset=0
  BogieSupportedMass : Inport  Port=4  Partition=on  PartitionDimension=1  PartitionWidth=1  PartitionOffset=0
  Reset : Inport  Port=5
  Faults : Inport  Port=6
  AirLevelingValve : Subsystem
  AirSuspensionReservoir : PneumaticLib/Limited Air Pressure Vessel  resetPrs=450000 + PAtm
      settings: SourceProductName=Pneumatic
  B27-L11-1/2 : PneumaticLib/Pressure Switch  OnSwitchValue=PressureSwitchON  OffSwitchValue=PressureSwitchOFF  OnOutputValue=1  OffOutputValue=0  InitOn=on
      settings: SourceProductName=Train Library
  Bias : Bias  Bias=-PAtm
  Bus Selector1 : BusSelector  OutputSignals=BECU1CarLoadPressureLow,BECU2CarLoadPressureLow,BECU1LoadPressureLow,AirSuspensionBogie1Deflated
  Constant : Constant  Value=PAtm + MaxPressure
  Constant1 : Constant  Value=true  OutDataTypeStr=boolean
  Display : Display
  FlowCalc : Subsystem
  For Each : ForEach  DisableCoverage=on
  NOT : Logic  Operator=NOT  AllPortsSameDT=off  OutDataTypeStr=boolean
  OR1 : Logic  Operator=OR  AllPortsSameDT=off  OutDataTypeStr=boolean
  OR2 : Logic  Operator=OR  Inputs=3  AllPortsSameDT=off  OutDataTypeStr=boolean
  Subsystem : Subsystem
  Terminator : Terminator
  Unit Delay : UnitDelay  SampleTime=-1  HasFrameUpgradeWarning=on
  Unit Delay1 : UnitDelay  SampleTime=-1  HasFrameUpgradeWarning=on
  Volume : Constant  Value=Volume
  pAtm : Constant  Value=PAtm
  AirSuspensionPressure : Outport  ConcatenationDimension=1
  AirSuspensionValve : Outport  Port=2  ConcatenationDimension=1
  AirSuspensionPressureSwitch : Outport  Port=3  ConcatenationDimension=1
  AirSuspPressure%Variation : Outport  Port=4  ConcatenationDimension=1
  ASRToAS : Outport  Port=5  ConcatenationDimension=1
  wires:
  Volume/1 -> AirSuspensionReservoir/2
  AirLevelingValve/1(TargetPressure) -> FlowCalc/3(TargetPressure), Subsystem/5(TargetPressure), AirSuspensionReservoir/7
  pAtm/1 -> AirSuspensionReservoir/4
  Reset/1 -> AirSuspensionReservoir/5
  Unit Delay/1 -> AirLevelingValve/1(AirSuspensionPressure), FlowCalc/2(AirSuspensionPressure)
  Constant/1 -> AirSuspensionReservoir/3
  FlowCalc/2(Flow) -> AirSuspensionReservoir/1
  AirSuspensionReservoir/2 -> Terminator/1
  AirSuspensionIsolCock/1 -> FlowCalc/5(AirSuspensionIsolCock)
  AirSuspensionDrainCock/1 -> FlowCalc/6(AirSuspensionDrainCock)
  AirLevelingValve/2(AirSuspensionValve) -> AirSuspensionValve/1, FlowCalc/4(AirSuspensionValve)
  NOT/1 -> AirSuspensionReservoir/6
  Unit Delay1/1 -> NOT/1
  Constant1/1 -> Unit Delay1/1
  Bias/1 -> B27-L11-1/2/1, Display/1
  B27-L11-1/2/1 -> AirSuspensionPressureSwitch/1
  BogieSupportedMass/1 -> AirLevelingValve/3(BogieSupportedMass)
  Bus Selector1/1 -> OR1/1  "<BECU1CarLoadPressureLow>"
  Bus Selector1/2 -> OR1/2  "<BECU2CarLoadPressureLow>"
  Faults/1 -> Bus Selector1/1
  AirSuspensionSupplyPressure/1 -> FlowCalc/1(AirSuspensionSupplyPressure)
  OR1/1 -> OR2/1, Subsystem/1(CarLoadPressureLow)
  Subsystem/1(PressureOut) -> AirSuspensionPressure/1, Bias/1, Unit Delay/1
  Bus Selector1/3 -> OR2/2, Subsystem/2(<BECU1LoadPressureLow>)  "<BECU1LoadPressureLow>"
  Bus Selector1/4 -> Subsystem/3(<AirSuspensionBogie1Deflated>), OR2/3  "<AirSuspensionBogie1Deflated>"
  OR2/1 -> AirLevelingValve/2(LoadPressureAbnormal)
  AirSuspensionReservoir/1 -> Subsystem/4(Pressure)
  Subsystem/2(AirSuspPressure%Variation) -> AirSuspPressure%Variation/1
  FlowCalc/1(ASRToAS) -> ASRToAS/1

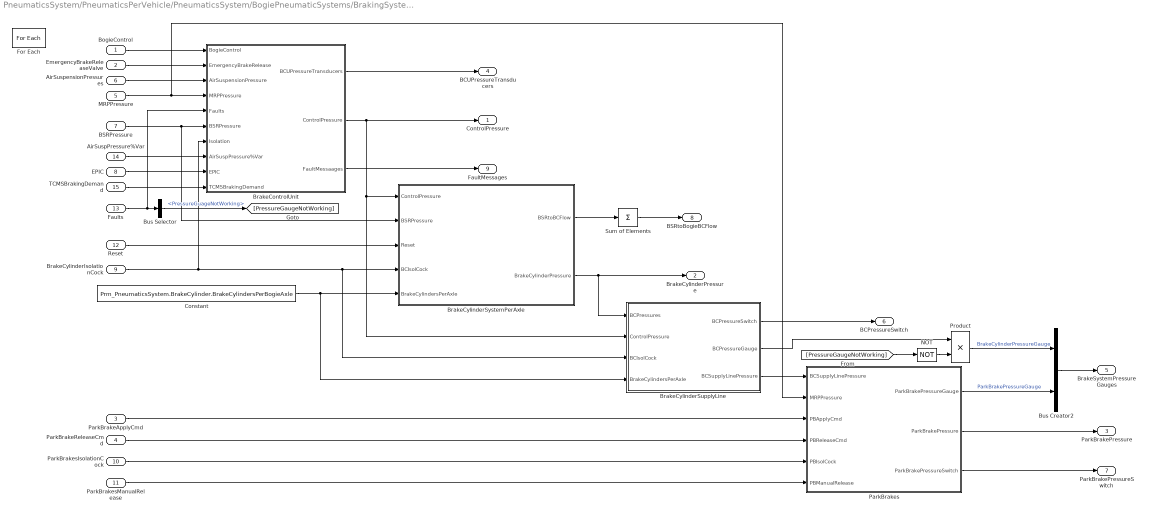
== system PneumaticsSystem/PneumaticsPerVehicle/PneumaticsSystem/BogiePneumaticSystems/BrakingSystem/BrakingSystemPerBogie ==
  BogieControl : Inport  Partition=on  PartitionDimension=1  PartitionWidth=1  PartitionOffset=0
  EmergencyBrakeReleaseValve : Inport  Port=2
  ParkBrakeApplyCmd : Inport  Port=3
  ParkBrakeReleaseCmd : Inport  Port=4
  MRPPressure : Inport  Port=5
  "AirSuspensionPressures " : Inport  Port=6  Partition=on  PartitionDimension=1  PartitionWidth=1  PartitionOffset=0
  BSRPressure : Inport  Port=7
  EPIC : Inport  Port=8
  BrakeCylinderIsolationCock : Inport  Port=9  Partition=on  PartitionDimension=1  PartitionWidth=1  PartitionOffset=0
  ParkBrakesIsolationCock : Inport  Port=10  Partition=on  PartitionDimension=1  PartitionWidth=1  PartitionOffset=0
  ParkBrakesManualRelease : Inport  Port=11  Partition=on  PartitionDimension=1  PartitionWidth=1  PartitionOffset=0
  Reset : Inport  Port=12
  Faults : Inport  Port=13
  AirSuspPressure%Var : Inport  Port=14  Partition=on  PartitionDimension=1  PartitionWidth=1  PartitionOffset=0
  TCMSBrakingDemand : Inport  Port=15
  BrakeControlUnit : Subsystem  mask{LoadCompensationPressures=Prm_PneumaticsSystem.AirSuspension.LoadCompensationPressures, LoadCompensationGains=Prm_PneumaticsSystem.BrakeControl.LoadCompensationGains, MaxControlPressure=Prm_PneumaticsSystem.BrakeControl.MaxPressure}
      mask prompts: LoadCompensationPressures "Load Compensation Pressures [Pa]"; LoadCompensationGains "Load Compensation Braking Gains [-]"; MaxControlPressure "Brake Control Max Pressure [Pa]"
  BrakeCylinderSupplyLine : Subsystem  mask{PressureSwitchON=Prm_PneumaticsSystem.BrakeCylinder.SwitchONPressure, PressureSwitchOFF=Prm_PneumaticsSystem.BrakeCylinder.SwitchOFFPressure}
      mask prompts: PressureSwitchON "Pressure Swith ON Point [Pa]"; PressureSwitchOFF "Pressure Swith OFF Point [Pa]"
  BrakeCylinderSystemPerAxle : Subsystem  mask{ResetPressure=Prm_PneumaticsSystem.BrakeCylinder.ResetPressure, MaxPressure=Prm_PneumaticsSystem.BrakeCylinder.MaxPressure, Volume=Prm_PneumaticsSystem.BrakeCylinder.Volume}
      mask prompts: ResetPressure "Reset Pressure [Pa]"; MaxPressure "Max Pressure [Pa]"; Volume "Cylinder Volume [m^3]"
      mask DialogControl Container10 Prompt: Brake Cylinder
  Bus Creator2 : BusCreator  Inputs=2  OutDataTypeStr=Bus: BD_PneumaticsSystem_Out_Vehicle_Gauges_Bogie  NonVirtualBus=on
  Bus Selector : BusSelector  OutputSignals=PressureGuageNotWorking
  Constant : Constant  Value=Prm_PneumaticsSystem.BrakeCylinder.BrakeCylindersPerBogieAxle
  For Each : ForEach  DisableCoverage=on
  NOT : Logic  Operator=NOT  AllPortsSameDT=off  OutDataTypeStr=boolean
  ParkBrakes : Subsystem  mask{AxleParkBrakeConfig=Prm_PneumaticsSystem.ParkBrakes.ParkBrakesPerBogieAxle, ParkingPressures=Prm_PneumaticsSystem.ParkBrakes.ParkBrakePressures, ParkingForces=Prm_PneumaticsSystem.ParkBrakes.ParkBrakeForces, PressureSwitchON=Prm_PneumaticsSystem.ParkBrakes.SwitchONPressure, PressureSwitchOFF=Prm_PneumaticsSystem.ParkBrakes.SwitchOFFPressure}
      mask prompts: AxleParkBrakeConfig "Bogie Configuration (0/1 per axle not/equipped)"; ParkingPressures "Park Brake Pressures (min and max) [Pa]"; ParkingForces "Park Braking Forces (Corresponding to min and max Pressures) [N]"; PressureSwitchON "Pressure Switch ON Point [Pa]"; PressureSwitchOFF "Pressure Switch OFF Point [Pa]"
      mask DialogControl ParameterGroupVar Prompt: Park Brakes Parameters
  Product : Product
  Sum of Elements : Sum  Inputs=+
  ControlPressure : Outport  ConcatenationDimension=1
  BrakeCylinderPressure : Outport  Port=2  ConcatenationDimension=1
  ParkBrakePressure : Outport  Port=3  ConcatenationDimension=1
  BCUPressureTransducers : Outport  Port=4  ConcatenationDimension=1
  BrakeSystemPressureGauges : Outport  Port=5  ConcatenationDimension=1
  BCPressureSwitch : Outport  Port=6  ConcatenationDimension=1
  ParkBrakePressureSwitch : Outport  Port=7  ConcatenationDimension=1
  BSRtoBogieBCFlow : Outport  Port=8  ConcatenationDimension=1
  FaultMessages : Outport  Port=9  ConcatenationDimension=1
  wires:
  BogieControl/1 -> BrakeControlUnit/1(BogieControl)
  BSRPressure/1 -> BrakeControlUnit/6(BSRPressure), BrakeCylinderSystemPerAxle/2(BSRPressure)
  EmergencyBrakeReleaseValve/1 -> BrakeControlUnit/2(EmergencyBrakeRelease)
  "AirSuspensionPressures "/1 -> BrakeControlUnit/3(AirSuspensionPressure)
  MRPPressure/1 -> BrakeControlUnit/4(MRPPressure), ParkBrakes/2(MRPPressure)
  BrakeControlUnit/2(ControlPressure) -> BrakeCylinderSupplyLine/2(ControlPressure), BrakeCylinderSystemPerAxle/1(ControlPressure), ControlPressure/1
  BrakeControlUnit/1(BCUPressureTransducers) -> BCUPressureTransducers/1
  Constant/1 -> BrakeCylinderSupplyLine/4(BrakeCylindersPerAxle), BrakeCylinderSystemPerAxle/5(BrakeCylindersPerAxle)
  BrakeCylinderIsolationCock/1 -> BrakeControlUnit/7(Isolation), BrakeCylinderSupplyLine/3(BCIsolCock), BrakeCylinderSystemPerAxle/4(BCIsolCock)
  Reset/1 -> BrakeCylinderSystemPerAxle/3(Reset)
  BrakeCylinderSystemPerAxle/2(BrakeCylinderPressure) -> BrakeCylinderPressure/1, BrakeCylinderSupplyLine/1(BCPressures)
  BrakeCylinderSystemPerAxle/1(BSRtoBCFlow) -> Sum of Elements/1
  BrakeCylinderSupplyLine/3(BCSupplyLinePressure) -> ParkBrakes/1(BCSupplyLinePressure)
  ParkBrakesIsolationCock/1 -> ParkBrakes/5(PBIsolCock)
  BrakeCylinderSupplyLine/1(BCPressureSwitch) -> BCPressureSwitch/1
  Product/1 -> Bus Creator2/1  "BrakeCylinderPressureGauge"
  ParkBrakes/2(ParkBrakePressure) -> ParkBrakePressure/1
  ParkBrakes/3(ParkBrakePressureSwitch) -> ParkBrakePressureSwitch/1
  ParkBrakes/1(ParkBrakePressureGauge) -> Bus Creator2/2  "ParkBrakePressureGauge"
  Sum of Elements/1 -> BSRtoBogieBCFlow/1
  Bus Creator2/1 -> BrakeSystemPressureGauges/1
  ParkBrakesManualRelease/1 -> ParkBrakes/6(PBManualRelease)
  ParkBrakeApplyCmd/1 -> ParkBrakes/3(PBApplyCmd)
  ParkBrakeReleaseCmd/1 -> ParkBrakes/4(PBReleaseCmd)
  Faults/1 -> BrakeControlUnit/5(Faults), Bus Selector/1
  NOT/1 -> Product/2
  BrakeCylinderSupplyLine/2(BCPressureGauge) -> Product/1
  Bus Selector/1 -> [PressureGaugeNotWorking]  "<PressureGuageNotWorking>"
  [PressureGaugeNotWorking] -> NOT/1
  BrakeControlUnit/3(FaultMessaages) -> FaultMessages/1
  AirSuspPressure%Var/1 -> BrakeControlUnit/8(AirSuspPressure%Var)
  EPIC/1 -> BrakeControlUnit/9(EPIC)
  TCMSBrakingDemand/1 -> BrakeControlUnit/10(TCMSBrakingDemand)

== system PneumaticsSystem/PneumaticsPerVehicle/PneumaticsSystem/BogiePneumaticSystems/SandingSystem/SandingSystemPerBogie ==
  SandingSystemIsolationCock : Inport  Partition=on  PartitionDimension=1  PartitionWidth=1  PartitionOffset=0
  SandingSystemSupplyPressure : Inport  Port=2
  SandingValve : Inport  Port=3
  Bias : Bias  Bias=-PAtm
  Divide : Product  Inputs=**
  Divide1 : Product  Inputs=**
  For Each : ForEach  DisableCoverage=on
  SandingPressureSwitch.10 : PneumaticLib/Pressure Switch  OnSwitchValue=PressureSwitchON  OffSwitchValue=PressureSwitchOFF  OnOutputValue=1  OffOutputValue=0  InitOn=on
      settings: SourceProductName=Train Library
  SandingPressure : Outport  ConcatenationDimension=1
  SandingPressureSwitch : Outport  Port=2  ConcatenationDimension=1
  wires:
  SandingSystemIsolationCock/1 -> Divide/1
  SandingPressureSwitch.10/1 -> Divide1/1
  Divide/1 -> SandingPressure/1, Bias/1  "SandingPressure"
  Bias/1 -> SandingPressureSwitch.10/1
  Divide1/1 -> SandingPressureSwitch/1  "SandingPressureSwitch"
  SandingValve/1 -> Divide1/2
  SandingSystemSupplyPressure/1 -> Divide/2

== system PneumaticsSystem/PneumaticsPerVehicle/PneumaticsSystem/BrakeReservoirSystem/BrakeSupplyReservoir/FlowCalc ==
  MRPressure : Inport
  BSRPressure : Inport  Port=2
  BSRIsolCock : Inport  Port=3
  BSRDrainCock : Inport  Port=4
  BSRtoBCFlow : Inport  Port=5
  Fault : Inport  Port=6
  Add : Sum  Inputs=+---
  BSR Charge : PneumaticLib/SS One Way Valve  d=0.015  p_deadband=1000
      settings: SourceProductName=Train Library
  BSR Vent Drain : PneumaticLib/SS One Way Valve  d=0.015  p_deadband=1000
      settings: SourceProductName=Train Library
  BSR Vent IC : PneumaticLib/SS One Way Valve  d=0.015  p_deadband=1000
      settings: SourceProductName=Train Library
  Compare To Constant : simulink/Logic and Bit Operations/Compare To Constant  relop=>  const=880000  OutDataTypeStr=boolean
  Constant : Constant  Value=PAtm
  Logical Operator1 : Logic  Operator=NOT  AllPortsSameDT=off  OutDataTypeStr=boolean
  Logical Operator2 : Logic  Operator=NOT  AllPortsSameDT=off  OutDataTypeStr=boolean
  Logical Operator3 : Logic  Operator=NOT  AllPortsSameDT=off  OutDataTypeStr=boolean
  Logical Operator4 : Logic  AllPortsSameDT=off  OutDataTypeStr=boolean
  Terminator : Terminator
  Terminator1 : Terminator
  Terminator4 : Terminator
  MRPToBSR : Outport
  Flow : Outport  Port=2
  wires:
  BSR Charge/1 -> MRPToBSR/1, Add/1
  Add/1 -> Flow/1
  BSR Charge/2 -> Terminator/1
  BSR Vent IC/2 -> Terminator1/1
  BSR Vent IC/1 -> Add/2
  MRPressure/1 -> BSR Charge/1
  Constant/1 -> BSR Vent IC/2, BSR Vent Drain/2
  BSRIsolCock/1 -> Logical Operator1/1
  Logical Operator1/1 -> BSR Charge/3
  BSRPressure/1 -> BSR Vent Drain/1, BSR Vent IC/1, Compare To Constant/1, BSR Charge/2
  BSR Vent Drain/2 -> Terminator4/1
  BSR Vent Drain/1 -> Add/3
  BSRDrainCock/1 -> Logical Operator2/1
  BSRtoBCFlow/1 -> Add/4
  Logical Operator2/1 -> BSR Vent Drain/3
  Fault/1 -> Logical Operator4/1
  Compare To Constant/1 -> Logical Operator4/2
  Logical Operator3/1 -> BSR Vent IC/3
  Logical Operator4/1 -> Logical Operator3/1

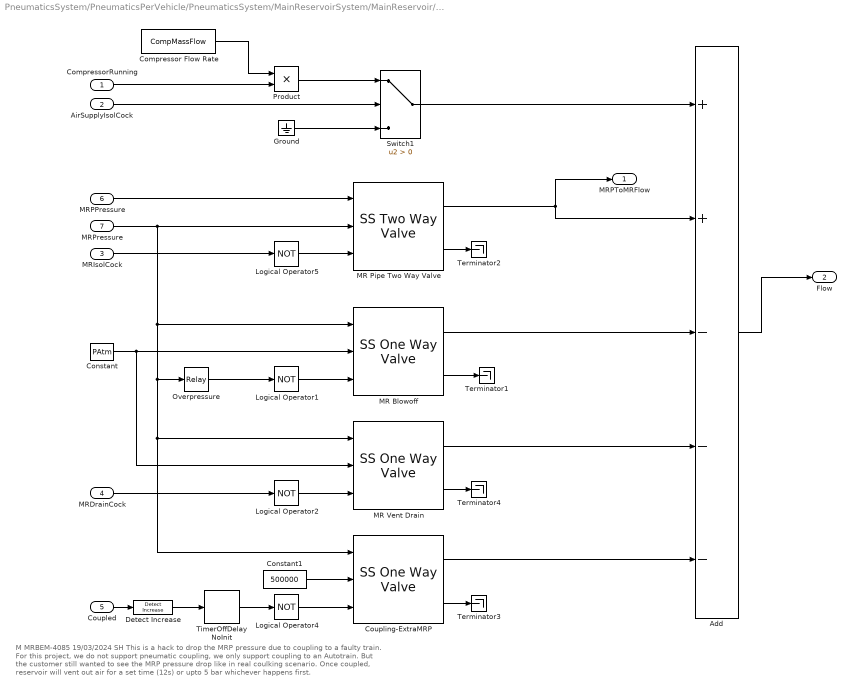
== system PneumaticsSystem/PneumaticsPerVehicle/PneumaticsSystem/MainReservoirSystem/MainReservoir/FlowCalc ==
  note: M MRBEM-4085 19/03/2024 SH
      | This is a hack to drop the MRP pressure due to coupling to a faulty train. For this project,
      | we do not support pneumatic coupling, we only support coupling to an Autotrain.
      | But the customer still wanted to see the MRP pressure drop like in real coulking scenario.
      | Once coupled, reservoir will vent out air for a set time (12s) or upto 5 bar whichever happens first.
  CompressorRunning : Inport
  AirSupplyIsolCock : Inport  Port=2
  MRIsolCock : Inport  Port=3
  MRDrainCock : Inport  Port=4
  Coupled : Inport  Port=5
  MRPPressure : Inport  Port=6
  MRPressure : Inport  Port=7
  Add : Sum  Inputs=++---
  Compressor Flow Rate : Constant  Value=CompMassFlow
  Constant : Constant  Value=PAtm
  Constant1 : Constant  Value=500000
  Coupling-ExtraMRP : PneumaticLib/SS One Way Valve  d=0.01  p_deadband=1000
      settings: SourceProductName=Train Library
  Detect Increase : simulink/Logic and Bit Operations/Detect Increase  vinit=0.0  OutDataTypeStr=boolean
  Ground : Ground
  Logical Operator{1..2,4..5} (4 alike) : Logic  Operator=NOT  AllPortsSameDT=off  OutDataTypeStr=boolean
  MR Blowoff : PneumaticLib/SS One Way Valve  d=0.01  p_deadband=1000
      settings: SourceProductName=Train Library
  MR Pipe Two Way Valve : PneumaticLib/SS Two Way Valve  d=0.01  p_deadband=1000
      settings: SourceProductName=Train Library
  MR Vent Drain : PneumaticLib/SS One Way Valve  d=0.01  p_deadband=1000
      settings: SourceProductName=Train Library
  Overpressure : Relay  OnSwitchValue=BlowOffON + PAtm  OffSwitchValue=BlowOffOFF + PAtm
  Product : Product
  Switch1 : Switch  Criteria=u2 > Threshold
  Terminator{1..4} (4 alike) : Terminator
  TimerOffDelay NoInit : TimersLib/TimerOffDelay NoInit  UpperSaturationLimit=12  SampleTime=-1
      settings: SourceProductName=Sydac Utilities
  MRPToMRFlow : Outport
  Flow : Outport  Port=2
  wires:
  Logical Operator2/1 -> MR Vent Drain/3
  MR Vent Drain/2 -> Terminator4/1
  Constant/1 -> MR Blowoff/2, MR Vent Drain/2
  MR Blowoff/2 -> Terminator1/1
  Add/1 -> Flow/1
  AirSupplyIsolCock/1 -> Switch1/2
  Overpressure/1 -> Logical Operator1/1
  Logical Operator1/1 -> MR Blowoff/3
  MRPPressure/1 -> MR Pipe Two Way Valve/1
  MRIsolCock/1 -> Logical Operator5/1
  MR Pipe Two Way Valve/2 -> Terminator2/1
  Switch1/1 -> Add/1
  MR Blowoff/1 -> Add/3
  MR Vent Drain/1 -> Add/4
  Logical Operator5/1 -> MR Pipe Two Way Valve/3
  MR Pipe Two Way Valve/1 -> MRPToMRFlow/1, Add/2
  Compressor Flow Rate/1 -> Product/1
  Product/1 -> Switch1/1
  Ground/1 -> Switch1/3
  CompressorRunning/1 -> Product/2
  MRDrainCock/1 -> Logical Operator2/1
  Coupled/1 -> Detect Increase/1
  Coupling-ExtraMRP/1 -> Add/5
  MRPressure/1 -> Coupling-ExtraMRP/1, MR Vent Drain/1, Overpressure/1, MR Blowoff/1, MR Pipe Two Way Valve/2
  Constant1/1 -> Coupling-ExtraMRP/2
  Coupling-ExtraMRP/2 -> Terminator3/1
  Logical Operator4/1 -> Coupling-ExtraMRP/3
  Detect Increase/1 -> TimerOffDelay NoInit/1
  TimerOffDelay NoInit/1 -> Logical Operator4/1
